simulink model "BrakeTest"  (R2024b)
settings: Solver=VariableStepAuto  StartTime=0.0  StopTime=1.5  RelTol=1e-3
undefined symbols (not defined in the file or in its folder): car
libraries: slpidlib x1, autolibshared x1
settings Model: Creator=franc  LastModifiedBy=franc

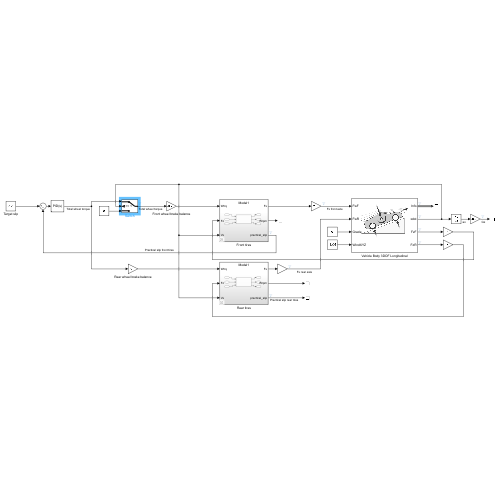
[thumbnail: Simulink's stored preview of the top-level diagram]
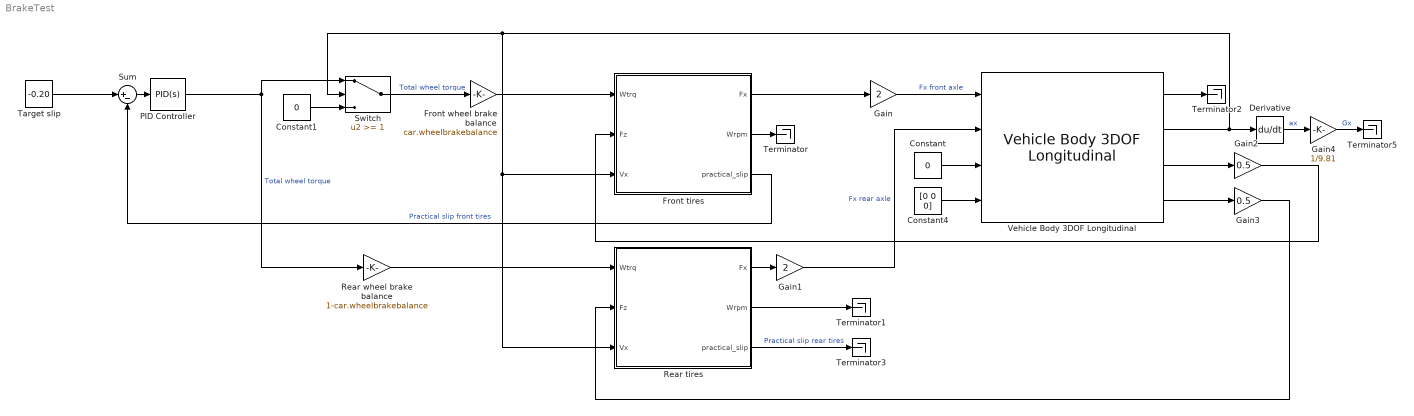
== system BrakeTest ==
  Constant : Constant  Value=0
  Constant1 : Constant  Value=0
  Constant4 : Constant  Value=[0 0 0]
  Derivative : Derivative
  Front tires : Subsystem  Variant=on
  Front wheel brake balance : Gain  Gain=car.wheelbrakebalance
  Gain : Gain  Gain=2
  Gain1 : Gain  Gain=2
  Gain2 : Gain  Gain=0.5
  Gain3 : Gain  Gain=0.5
  Gain4 : Gain  Gain=1/9.81
  PID Controller : slpidlib/PID Controller  Controller=PID  Form=Parallel  TimeDomain=Continuous-time  UseExternalTs=off  SampleTime=-1  IntegratorMethod=Forward Euler  FilterMethod=Forward Euler  ControllerParametersSource=internal  P=30000  I=10000  UseKiTs=off  D=1000  UseExternalDerivativeSource=off  N=100  UseFilter=on  TunerSelectOption=Transfer Function Based (PID Tuner App)  InitialConditionSource=internal  InitialConditionForIntegrator=0  InitialConditionForFilter=0  DifferentiatorICPrevScaledInput=0  ExternalReset=none  TrackingMode=off  Kt=1  LimitOutput=off  SatLimitsSource=internal  UpperSaturationLimit=inf  LowerSaturationLimit=-inf  LinearizeAsGain=on  AntiWindupMode=none  Kb=1  LimitIntegrator=off  UpperIntegratorSaturationLimit=inf  LowerIntegratorSaturationLimit=-inf  POutMin=[]  POutMax=[]  IOutMin=[]  IOutMax=[]  DOutMin=[]  DOutMax=[]  NOutMin=[]  NOutMax=[]  SumOutMin=[]  SumOutMax=[]  SaturationOutMin=[]  SaturationOutMax=[]  PParamMin=[]  PParamMax=[]  IParamMin=[]  IParamMax=[]  DParamMin=[]  DParamMax=[]  NParamMin=[]  NParamMax=[]  KbParamMin=[]  KbParamMax=[]  KtParamMin=[]  KtParamMax=[]  KbOutMin=[]  KbOutMax=[]  KtOutMin=[]  KtOutMax=[]  IntegratorOutMin=[]  IntegratorOutMax=[]  FilterOutMin=[]  FilterOutMax=[]  SumI1OutMin=[]  SumI1OutMax=[]  SumI2OutMin=[]  SumI2OutMax=[]  SumI3OutMin=[]  SumI3OutMax=[]  SumI4OutMin=[]  SumI4OutMax=[]  SumDOutMin=[]  SumDOutMax=[]  DifferentiatorOutMin=[]  DifferentiatorOutMax=[]  FilterDiffOutCoefMin=[]  FilterDiffOutCoefMax=[]  ReciprocalOutMin=[]  ReciprocalOutMax=[]  SumDenOutMin=[]  SumDenOutMax=[]  SumNumOutMin=[]  SumNumOutMax=[]  DivideOutMin=[]  DivideOutMax=[]  UdiffTsProdOutMin=[]  UdiffTsProdOutMax=[]  NTsProdOutMin=[]  NTsProdOutMax=[]  UintegralTsProdOutMin=[]  UintegralTsProdOutMax=[]  UngainTsProdOutMin=[]  UngainTsProdOutMax=[]  ClampingZeroOutDataTypeStr=Inherit: Inherit via back propagation  ClampingZeroOutMin=[]  ClampingZeroOutMax=[]  FilterDenConstantOutDataTypeStr=Inherit: Inherit via back propagation  FilterDenConstantOutMin=[]  FilterDenConstantOutMax=[]  PCopyOutDataTypeStr=Inherit: Inherit via back propagation  PCopyOutMin=[]  PCopyOutMax=[]  NCopyOutDataTypeStr=Inherit: Inherit via back propagation  NCopyOutMin=[]  NCopyOutMax=[]  IntegratorContinuousStateAttributes=''  IntegratorStateMustResolveToSignalObject=off  IntegratorRTWStateStorageClass=Auto  FilterContinuousStateAttributes=''  FilterStateMustResolveToSignalObject=off  FilterRTWStateStorageClass=Auto  ParallelPVariant=InternalParameters  IdealPVariant=Disabled  IVariant=InternalParameters  DVariant=InternalParameters  IntegratorVariant=Continuous  SatVariant=Disabled  AWVariant=Passthrough  PCopyVariant=Disabled  TRVariant=Disabled  FdbkBlocksVariant=Forward  IdealPFdbkVariant=Disabled  SatFdbkVariant=Disabled  DerivativeFilterVariant=ContFilter  NVariant=InternalParameters  NCopyVariant=Disabled  FilterICVariant=InternalICsFilter  IntegratorICVariant=InternalICs  ExternalResetVariant=Disabled  TRSumVariant=Passthrough  SumFdbkVariant=Disabled  SumVariant=Sum_PID  TsampFilterVariant=InternalTs  TsampNgainVariant=Passthrough  TsampIntegralVariant=Disabled_SignalSpec  ExternalSaturationOutDataTypeStr=Inherit: Same as second input  DerivativeSourceVariant=ErrorSignal  PreIntVariant=InternalPreInt
  Rear tires : Subsystem  Variant=on
  Rear wheel brake balance : Gain  Gain=1-car.wheelbrakebalance
  Sum : Sum  Inputs=|+-
  Switch : Switch  Threshold=1  SaturateOnIntegerOverflow=off  InputSameDT=off
  Target slip : Constant  Value=-0.20
  Terminator{,1..3,5} (5 alike) : Terminator
  Vehicle Body 3DOF Longitudinal : autolibshared/Vehicle Body 3DOF Longitudinal  VariantControl=SL  groundType=Grade angle  aMode=2  extFMode=off  extMMode=off  extTamb=off  NF=2  NR=2  m=car.Longitudinalbody.Mass  a=car.Longitudinalbody.COGa  b=car.Longitudinalbody.COGb  h=car.Longitudinalbody.COGh  Cd=car.Longitudinalbody.Cd  Af=car.Longitudinalbody.Af  x_o=0  xdot_o=car.Longitudinalbody.braketest.v0  Cl=car.Longitudinalbody.Cl  z_o=car.Longitudinalbody.COGz_o  zdot_o=0  Iyy=car.Longitudinalbody.I(2)  Cpm=.1  theta_o=0  q_o=0  FskF=car.Longitudinalbody.FskF  dzsF=car.Longitudinalbody.dzsF  FsbF=car.Longitudinalbody.FsbF  dzdotsF=car.Longitudinalbody.dzdotsF  FskR=car.Longitudinalbody.FskR  dzsR=car.Longitudinalbody.dzsR  FsbR=car.Longitudinalbody.FsbR  dzdotsR=car.Longitudinalbody.dzdotsR  Pabs=101325  T=273  g=9.81  blkID=0
      settings: LibrarySourceBlock=vehdynlibeom/Vehicle Body 3DOF Longitudinal
  wires:
  Front tires/1(Fx) -> Gain/1
  Rear tires/1(Fx) -> Gain1/1
  Gain/1 -> Vehicle Body 3DOF Longitudinal/1  "Fx front axle"
  Gain1/1 -> Vehicle Body 3DOF Longitudinal/2  "Fx rear axle"
  Front tires/2(Wrpm) -> Terminator/1
  Rear tires/2(Wrpm) -> Terminator1/1
  Constant/1 -> Vehicle Body 3DOF Longitudinal/3
  Constant4/1 -> Vehicle Body 3DOF Longitudinal/4
  Vehicle Body 3DOF Longitudinal/1 -> Terminator2/1
  Vehicle Body 3DOF Longitudinal/3 -> Gain2/1
  Vehicle Body 3DOF Longitudinal/4 -> Gain3/1
  Gain3/1 -> Rear tires/2(Fz)
  Gain2/1 -> Front tires/2(Fz)
  Vehicle Body 3DOF Longitudinal/2 -> Rear tires/3(Vx), Front tires/3(Vx), Switch/2, Derivative/1
  Rear tires/3(practical_slip) -> Terminator3/1  "Practical slip rear tires"
  PID Controller/1 -> Switch/1, Rear wheel brake balance/1  "Total wheel torque"
  Front wheel brake balance/1 -> Front tires/1(Wtrq)
  Rear wheel brake balance/1 -> Rear tires/1(Wtrq)
  Derivative/1 -> Gain4/1  "ax"
  Gain4/1 -> Terminator5/1  "Gx"
  Target slip/1 -> Sum/1
  Front tires/3(practical_slip) -> Sum/2  "Practical slip front tires"
  Sum/1 -> PID Controller/1
  Switch/1 -> Front wheel brake balance/1  "Total wheel torque"
  Constant1/1 -> Switch/3

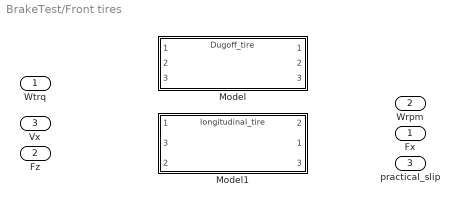
== system BrakeTest/Front tires ==
  Wtrq : Inport
  Fz : Inport  Port=2
  Vx : Inport  Port=3
  Model : ModelReference  DisableCoverage=on  ModelNameDialog=Dugoff_tire.slx  SimulationMode=Normal  VariantControl=false  ModelReferenceVersion=2.16
  Model1 : ModelReference  ModelNameDialog=longitudinal_tire.slx  SimulationMode=Normal  VariantControl=true  ModelReferenceVersion=3.7
      settings: PortSchema="{\"entries\":[{\"content\":{\"sides\":[{\"content\":{\"connectorIds\":[\"In1\",\"In3\",\"In2\"]},\"type\":\"ConnectorPlacement.EquallySpacedRectSide\",\"uuid\":\"5eba1a74-bd07-49e9-ac91-356b950fcd72\"},{\"content\":{\"connectorIds\":[\"Out2\",\"Out1\",\"Out3\"],\"side\":\"RIGHT\"},\"type\":\"ConnectorPlacement.EquallySpacedRectSide\",\"uuid\":\"1040ce78-c535-419a-aa8f-ad6fbf19e979\"},{\"content\":{\"side\":\"TOP\"},\"type\":\"ConnectorPlacement.EquallySpacedRectSide\",\"uuid\":\"ba0f3e1f-76c3-4461-91cd-c7f47b575855\"}]},\"type\":\"ConnectorPlacement.EquallySpacedConnector\",\"uuid\":\"77c71335-a5e7-4e66-a78b-88921c7c7d22\"}],\"packageUris\":[\"http://schema.mathworks.com/mf0/Connector/R2020b\"],\"version\":\"1.0\"}"
  Fx : Outport
  Wrpm : Outport  Port=2
  practical_slip : Outport  Port=3

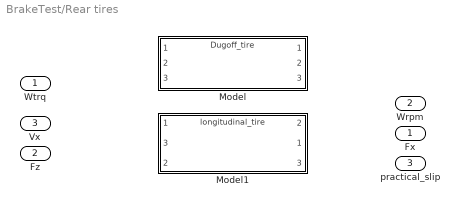
== system BrakeTest/Rear tires ==
  Wtrq : Inport
  Fz : Inport  Port=2
  Vx : Inport  Port=3
  Model : ModelReference  DisableCoverage=on  ModelNameDialog=Dugoff_tire.slx  SimulationMode=Normal  VariantControl=false  ModelReferenceVersion=2.16
  Model1 : ModelReference  ModelNameDialog=longitudinal_tire.slx  SimulationMode=Normal  VariantControl=true  ModelReferenceVersion=3.7
      settings: PortSchema="{\"entries\":[{\"content\":{\"sides\":[{\"content\":{\"connectorIds\":[\"In1\",\"In3\",\"In2\"]},\"type\":\"ConnectorPlacement.EquallySpacedRectSide\",\"uuid\":\"5eba1a74-bd07-49e9-ac91-356b950fcd72\"},{\"content\":{\"connectorIds\":[\"Out2\",\"Out1\",\"Out3\"],\"side\":\"RIGHT\"},\"type\":\"ConnectorPlacement.EquallySpacedRectSide\",\"uuid\":\"1040ce78-c535-419a-aa8f-ad6fbf19e979\"},{\"content\":{\"side\":\"TOP\"},\"type\":\"ConnectorPlacement.EquallySpacedRectSide\",\"uuid\":\"ba0f3e1f-76c3-4461-91cd-c7f47b575855\"}]},\"type\":\"ConnectorPlacement.EquallySpacedConnector\",\"uuid\":\"77c71335-a5e7-4e66-a78b-88921c7c7d22\"}],\"packageUris\":[\"http://schema.mathworks.com/mf0/Connector/R2020b\"],\"version\":\"1.0\"}"
  Fx : Outport
  Wrpm : Outport  Port=2
  practical_slip : Outport  Port=3
